simulink model "theta_x_PendulumInverseSIMU"  (Simulink 10.0)
settings: Solver=ode45  StartTime=ti  StopTime=tf  FixedStep=0.001  RelTol=1e-3  EnableMultiTasking=on
undefined symbols (not defined in the file): alpha, g, gain, J, l, m, Mcart, n, Noise, theta
libraries: simulink x1
settings Model: Creator=huojiaxi  LastModifiedBy=huojiaxi  ExtModeTrigMode=oneshot  ExtModeArmWhenConnect=off
settings DataIOCC: SignalLoggingSaveFormat=ModelDataLogs
settings OptimizationCC: BooleanDataType=off  LifeSpan=auto
settings DebuggingCC: SaveWithParameterizedLinksMsg=none  SignalResolutionControl=TryResolveAllWithWarning  MultiTaskDSMMsg=warning  MultiTaskCondExecSysMsg=none  SFUnexpectedBacktrackingDiag=error  SFNoUnconditionalDefaultTransitionDiag=error  SFExecutionAtInitializationDiag=warning  ArithmeticOperatorsInVariantConditions=error
settings HardwareCC: ProdBitPerPointer=64  ProdBitPerSizeT=64  ProdBitPerPtrDiffT=64  ProdLargestAtomicFloat=Float  ProdIntDivRoundTo=Zero  ProdEndianess=LittleEndian  ProdWordSize=64  ProdHWDeviceType=Intel->x86-64 (Windows64)  TargetUnknown=on
settings SFSimCC: SimUseLocalCustomCode=on  CustomCodeUndefinedFunction=FilterOut
settings RTWCC: RTWUseLocalCustomCode=on
settings CodeAppCC: StateflowObjectComments=off
settings GRTTargetCC: TargetLangStandard=C99 (ISO)
settings ConfigComp: CovSaveCumulativeToWorkspaceVar=off  CovSaveSingleToWorkspaceVar=off

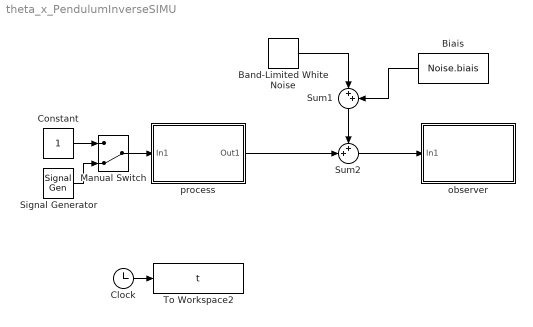
== system theta_x_PendulumInverseSIMU ==
  Band-Limited White Noise : simulink/Sources/Band-Limited White Noise  Cov=Noise.power  Ts=Noise.sampling  seed=Noise.seed
  Biais : Constant  Value=Noise.biais
  Clock : Clock
  Constant : Constant
  Manual Switch : ManualSwitch  CurrentSetting=0
  Signal Generator : SignalGenerator  Units=rad/sec
  Sum1 : Sum  Inputs=|++
  Sum2 : Sum  Inputs=++|
  To Workspace2 : ToWorkspace  VariableName=t  SampleTime=-1
  observer : Subsystem
  process : Subsystem
  wires:
  Sum1/1 -> Sum2/1
  Biais/1 -> Sum1/2
  Band-Limited White Noise/1 -> Sum1/1
  Sum2/1 -> observer/1(In1)
  process/1(Out1) -> Sum2/2
  Clock/1 -> To Workspace2/1
  Manual Switch/1 -> process/1(In1)
  Constant/1 -> Manual Switch/1
  Signal Generator/1 -> Manual Switch/2

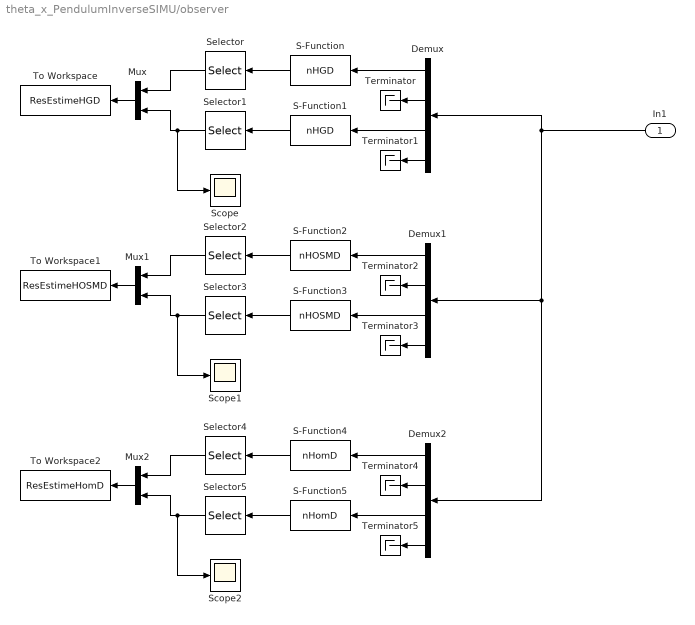
== system theta_x_PendulumInverseSIMU/observer ==
  In1 : Inport
  Demux : Demux
  Demux1 : Demux
  Demux2 : Demux
  Mux : Mux  Inputs=2
  Mux1 : Mux  Inputs=2
  Mux2 : Mux  Inputs=2
  S-Function : S-Function  FunctionName=nHGD  Parameters=n,gain,theta  SFunctionDeploymentMode=off  EnableBusSupport=off
  S-Function1 : S-Function  FunctionName=nHGD  Parameters=n,gain,theta  SFunctionDeploymentMode=off  EnableBusSupport=off
  S-Function2 : S-Function  FunctionName=nHOSMD  Parameters=n,gain,theta  SFunctionDeploymentMode=off  EnableBusSupport=off
  S-Function3 : S-Function  FunctionName=nHOSMD  Parameters=n,gain,theta  SFunctionDeploymentMode=off  EnableBusSupport=off
  S-Function4 : S-Function  FunctionName=nHomD  Parameters=n,gain,theta,alpha  SFunctionDeploymentMode=off  EnableBusSupport=off
  S-Function5 : S-Function  FunctionName=nHomD  Parameters=n,gain,theta,alpha  SFunctionDeploymentMode=off  EnableBusSupport=off
  Scope : Scope
  Scope1 : Scope
  Scope2 : Scope
  Selector{,1..5} (6 alike) : Selector  InputPortWidth=n+1  IndexOptions=Index vector (dialog)  Indices=[1 2]  OutputSizes=1
  Terminator{,1..5} (6 alike) : Terminator
  To Workspace : ToWorkspace  VariableName=ResEstimeHGD  SampleTime=-1
  To Workspace1 : ToWorkspace  VariableName=ResEstimeHOSMD  SampleTime=-1
  To Workspace2 : ToWorkspace  VariableName=ResEstimeHomD  SampleTime=-1
  wires:
  Demux/3 -> S-Function1/1
  Demux/4 -> Terminator1/1
  Selector1/1 -> Mux/2, Scope/1
  Demux/1 -> S-Function/1
  Selector/1 -> Mux/1
  S-Function1/1 -> Selector1/1
  S-Function/1 -> Selector/1
  Demux/2 -> Terminator/1
  Mux/1 -> To Workspace/1
  Demux1/3 -> S-Function3/1
  Demux1/2 -> Terminator2/1
  Demux1/1 -> S-Function2/1
  Mux1/1 -> To Workspace1/1
  Selector2/1 -> Mux1/1
  Selector3/1 -> Mux1/2, Scope1/1
  S-Function2/1 -> Selector2/1
  S-Function3/1 -> Selector3/1
  Demux1/4 -> Terminator3/1
  Demux2/3 -> S-Function5/1
  In1/1 -> Demux2/1, Demux1/1, Demux/1
  Demux2/2 -> Terminator4/1
  Demux2/1 -> S-Function4/1
  Mux2/1 -> To Workspace2/1
  Selector4/1 -> Mux2/1
  Selector5/1 -> Mux2/2, Scope2/1
  S-Function4/1 -> Selector4/1
  S-Function5/1 -> Selector5/1
  Demux2/4 -> Terminator5/1

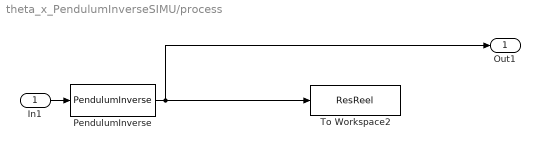
== system theta_x_PendulumInverseSIMU/process ==
  In1 : Inport
  PendulumInverse : S-Function  FunctionName=PendulumInverse  Parameters=Mcart,m,l,g,J  SFunctionDeploymentMode=off  EnableBusSupport=off
  To Workspace2 : ToWorkspace  VariableName=ResReel  SampleTime=-1
  Out1 : Outport
  wires:
  In1/1 -> PendulumInverse/1
  PendulumInverse/1 -> To Workspace2/1, Out1/1
